simulink model "minimum_snap_trajectory"  (R2021a)
settings: Solver=VariableStepAuto  StartTime=0.0  StopTime=T_s  RelTol=1e-3
values from neighbouring files (symbols this model uses):
  a_x = x(1,1:(length(x)-1))    [Linearized_model.m]    (also in Linearized_model_motor_dynamics.m)
  a_y = y(1,1:(length(y)-1))    [Linearized_model.m]    (also in Linearized_model_motor_dynamics.m)
  a_z = z(1,1:(length(z)-1))    [Linearized_model.m]    (also in Linearized_model_motor_dynamics.m)
  b_x = x(1,2:length(x))    [Linearized_model.m]    (also in Linearized_model_motor_dynamics.m)
  b_y = y(1,2:length(y))    [Linearized_model.m]    (also in Linearized_model_motor_dynamics.m)
  b_z = z(1,2:length(z))    [Linearized_model.m]    (also in Linearized_model_motor_dynamics.m)
  T_r = zeros(1, length(T))    [Linearized_model.m]    (also in Linearized_model_motor_dynamics.m)
  T_s = sum(T)    [Linearized_model.m]    (also in Linearized_model_motor_dynamics.m)
undefined symbols (not defined in the file or in its folder): a_phi, a_si, a_theta, b_phi, b_si, b_theta
settings Model: Creator=Traveler  LastModifiedBy=Traveler

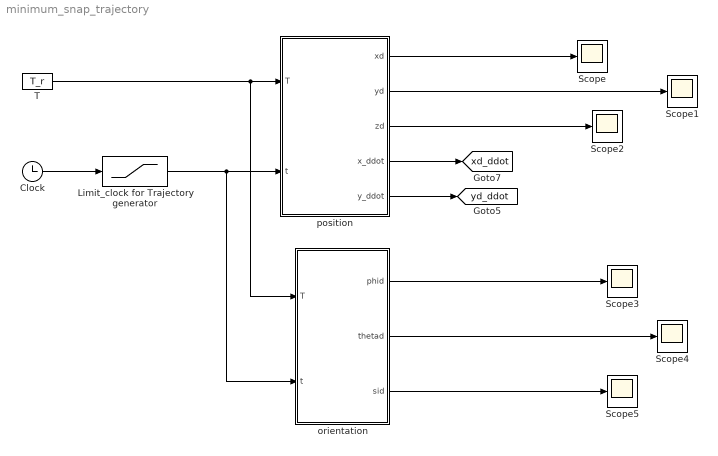
== system minimum_snap_trajectory ==
  Clock : Clock
  Limit_clock for Trajectory generator : Saturate  UpperLimit=T_s  LowerLimit=0
  Scope{,1..5} (6 alike) : Scope
  T : Constant  Value=T_r
  orientation : Subsystem
  position : Subsystem
  tag scope: xd_ddot=global, yd_ddot=global
  wires:
  position/5(y_ddot) -> [yd_ddot]
  T/1 -> orientation/1(T), position/1(T)
  Clock/1 -> Limit_clock for Trajectory generator/1
  orientation/2(thetad) -> Scope4/1
  position/2(yd) -> Scope1/1
  Limit_clock for Trajectory generator/1 -> orientation/2(t), position/2(t)
  position/3(zd) -> Scope2/1
  position/1(xd) -> Scope/1
  position/4(x_ddot) -> [xd_ddot]
  orientation/1(phid) -> Scope3/1
  orientation/3(sid) -> Scope5/1

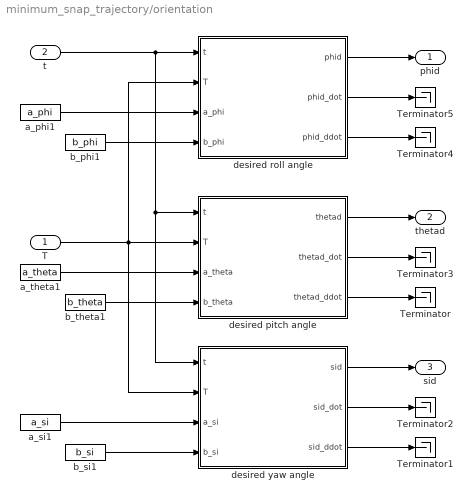
== system minimum_snap_trajectory/orientation ==
  T : Inport
  t : Inport  Port=2
  " desired pitch angle" : MATLAB Function  TreatAsAtomicUnit=on
  Terminator{,1..5} (6 alike) : Terminator
  a_phi1 : Constant  Value=a_phi
  a_si1 : Constant  Value=a_si
  a_theta1 : Constant  Value=a_theta
  b_phi1 : Constant  Value=b_phi
  b_si1 : Constant  Value=b_si
  b_theta1 : Constant  Value=b_theta
  desired roll angle : MATLAB Function  TreatAsAtomicUnit=on
  desired yaw angle : MATLAB Function  TreatAsAtomicUnit=on
  phid : Outport
  thetad : Outport  Port=2
  sid : Outport  Port=3
  wires:
  desired roll angle/1(phid) -> phid/1
  desired roll angle/2(phid_dot) -> Terminator5/1
  desired roll angle/3(phid_ddot) -> Terminator4/1
  " desired pitch angle"/3(thetad_ddot) -> Terminator/1
  " desired pitch angle"/2(thetad_dot) -> Terminator3/1
  " desired pitch angle"/1(thetad) -> thetad/1
  desired yaw angle/1(sid) -> sid/1
  desired yaw angle/2(sid_dot) -> Terminator2/1
  desired yaw angle/3(sid_ddot) -> Terminator1/1
  a_phi1/1 -> desired roll angle/3(a_phi)
  b_phi1/1 -> desired roll angle/4(b_phi)
  a_theta1/1 -> " desired pitch angle"/3(a_theta)
  b_theta1/1 -> " desired pitch angle"/4(b_theta)
  a_si1/1 -> desired yaw angle/3(a_si)
  b_si1/1 -> desired yaw angle/4(b_si)
  T/1 -> desired roll angle/2(T), " desired pitch angle"/2(T), desired yaw angle/2(T)
  t/1 -> desired yaw angle/1(t), " desired pitch angle"/1(t), desired roll angle/1(t)

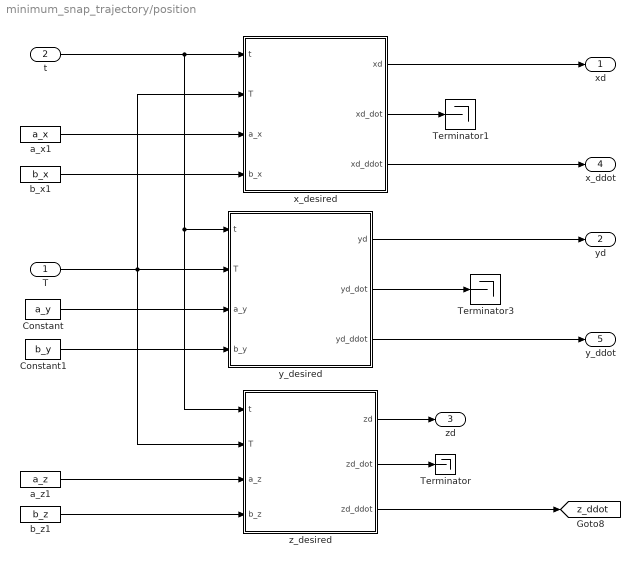
== system minimum_snap_trajectory/position ==
  T : Inport
  t : Inport  Port=2
  " z_desired" : MATLAB Function  TreatAsAtomicUnit=on
  Constant : Constant  Value=a_y
  Constant1 : Constant  Value=b_y
  Terminator : Terminator
  Terminator1 : Terminator
  Terminator3 : Terminator
  a_x1 : Constant  Value=a_x
  a_z1 : Constant  Value=a_z
  b_x1 : Constant  Value=b_x
  b_z1 : Constant  Value=b_z
  x_desired : MATLAB Function  TreatAsAtomicUnit=on
  y_desired : MATLAB Function  TreatAsAtomicUnit=on
  xd : Outport
  yd : Outport  Port=2
  zd : Outport  Port=3
  x_ddot : Outport  Port=4
  y_ddot : Outport  Port=5
  tag scope: z_ddot=global
  wires:
  y_desired/1(yd) -> yd/1
  T/1 -> x_desired/2(T), y_desired/2(T), " z_desired"/2(T)
  a_x1/1 -> x_desired/3(a_x)
  b_x1/1 -> x_desired/4(b_x)
  Constant/1 -> y_desired/3(a_y)
  Constant1/1 -> y_desired/4(b_y)
  a_z1/1 -> " z_desired"/3(a_z)
  b_z1/1 -> " z_desired"/4(b_z)
  " z_desired"/2(zd_dot) -> Terminator/1
  x_desired/2(xd_dot) -> Terminator1/1
  y_desired/2(yd_dot) -> Terminator3/1
  t/1 -> x_desired/1(t), y_desired/1(t), " z_desired"/1(t)
  " z_desired"/3(zd_ddot) -> [z_ddot]
  " z_desired"/1(zd) -> zd/1
  y_desired/3(yd_ddot) -> y_ddot/1
  x_desired/3(xd_ddot) -> x_ddot/1
  x_desired/1(xd) -> xd/1

== matlab function minimum_snap_trajectory/orientation/ desired pitch angle ==
  data: t input; T input; thetad output; thetad_dot output; thetad_ddot output; a_theta input; b_theta input
function [thetad,thetad_dot,thetad_ddot] = fcn(t,T,a_theta,b_theta)
T0 = 0; % Initialize T0
Tf = 0; % Initialize Tf
a = 0;  % Initialize a
b = 0;  % Initialize b

for i = 1:length(T)
    if (i == 1 && t <= T(i))
        Tf = T(i);
        a = a_theta(i);
        b = b_theta(i);
        break;
    elseif (i > 1 && t > T(i-1) && t <= T(i))
        T0 = T(i-1);
        Tf = T(i);
        a = a_theta(i);
        b = b_theta(i);
        break;
    end
end
if (t > T(end-1)) % Handle the case where t is greater than the last interval
    T0 = T(end-1);
    Tf = T(end);
    a = a_theta(end);
    b = b_theta(end);
end
B=[a;b;0;0;0;0];
A=[T0^5     T0^4     T0^3    T0^2  T0^1  1;
   Tf^5     Tf^4     Tf^3    Tf^2  Tf^1  1;
   5*T0^4   4*T0^3   3*T0^2  2*T0  1     0;
   5*Tf^4   4*Tf^3   3*Tf^2  2*Tf  1     0;
   20*T0^3  12*T0^2  6*T0    2     0     0;
   20*Tf^3  12*Tf^2  6*Tf    2     0     0];
C=A\B;
thetad=C(1,1)*t^5 + C(2,1)*t^4 + C(3,1)*t^3 + C(4,1)*t^2 + C(5,1)*t + C(6,1);
thetad_dot=5*C(1,1)*t^4  + 4*C(2,1)*t^3 + 3*C(3,1)*t^2 + 2*C(4,1)*t + C(5,1);
thetad_ddot=20*C(1,1)*t^3  + 12*C(2,1)*t^2 + 6*C(3,1)*t + 2*C(4,1);
end

== matlab function minimum_snap_trajectory/orientation/desired roll angle ==
  data: t input; T input; phid output; phid_dot output; phid_ddot output; a_phi input; b_phi input
function [phid,phid_dot,phid_ddot] = fcn(t,T,a_phi,b_phi)
T0 = 0; % Initialize T0
Tf = 0; % Initialize Tf
a = 0;  % Initialize a
b = 0;  % Initialize b

for i = 1:length(T)
    if (i == 1 && t <= T(i))
        Tf = T(i);
        a = a_phi(i);
        b = b_phi(i);
        break;
    elseif (i > 1 && t > T(i-1) && t <= T(i))
        T0 = T(i-1);
        Tf = T(i);
        a = a_phi(i);
        b = b_phi(i);
        break;
    end
end
if (t > T(end-1)) % Handle the case where t is greater than the last interval
    T0 = T(end-1);
    Tf = T(end);
    a = a_phi(end);
    b = b_phi(end);
end
B=[a;b;0;0;0;0];
A=[T0^5     T0^4     T0^3    T0^2  T0^1  1;
   Tf^5     Tf^4     Tf^3    Tf^2  Tf^1  1;
   5*T0^4   4*T0^3   3*T0^2  2*T0  1     0;
   5*Tf^4   4*Tf^3   3*Tf^2  2*Tf  1     0;
   20*T0^3  12*T0^2  6*T0    2     0     0;
   20*Tf^3  12*Tf^2  6*Tf    2     0     0];
C=A\B;
phid=C(1,1)*t^5 + C(2,1)*t^4 + C(3,1)*t^3 + C(4,1)*t^2 + C(5,1)*t + C(6,1);
phid_dot=5*C(1,1)*t^4  + 4*C(2,1)*t^3 + 3*C(3,1)*t^2 + 2*C(4,1)*t + C(5,1);
phid_ddot=20*C(1,1)*t^3  + 12*C(2,1)*t^2 + 6*C(3,1)*t + 2*C(4,1);
end

== matlab function minimum_snap_trajectory/orientation/desired yaw angle ==
  data: t input; T input; sid output; sid_dot output; sid_ddot output; a_si input; b_si input
function [sid,sid_dot,sid_ddot] = fcn(t,T,a_si,b_si)
T0 = 0; % Initialize T0
Tf = 0; % Initialize Tf
a = 0;  % Initialize a
b = 0;  % Initialize b

for i = 1:length(T)
    if (i == 1 && t <= T(i))
        Tf = T(i);
        a = a_si(i);
        b = b_si(i);
        break;
    elseif (i > 1 && t > T(i-1) && t <= T(i))
        T0 = T(i-1);
        Tf = T(i);
        a = a_si(i);
        b = b_si(i);
        break;
    end
end
if (t > T(end-1)) % Handle the case where t is greater than the last interval
    T0 = T(end-1);
    Tf = T(end);
    a = a_si(end);
    b = b_si(end);
end
B=[a;b;0;0;0;0];
A=[T0^5     T0^4     T0^3    T0^2  T0^1  1;
   Tf^5     Tf^4     Tf^3    Tf^2  Tf^1  1;
   5*T0^4   4*T0^3   3*T0^2  2*T0  1     0;
   5*Tf^4   4*Tf^3   3*Tf^2  2*Tf  1     0;
   20*T0^3  12*T0^2  6*T0    2     0     0;
   20*Tf^3  12*Tf^2  6*Tf    2     0     0];
C=A\B;
sid=C(1,1)*t^5 + C(2,1)*t^4 + C(3,1)*t^3 + C(4,1)*t^2 + C(5,1)*t + C(6,1);
sid_dot=5*C(1,1)*t^4  + 4*C(2,1)*t^3 + 3*C(3,1)*t^2 + 2*C(4,1)*t + C(5,1);
sid_ddot=20*C(1,1)*t^3  + 12*C(2,1)*t^2 + 6*C(3,1)*t + 2*C(4,1);
end

== matlab function minimum_snap_trajectory/position/ z_desired ==
  data: t input; T input; zd output; zd_dot output; zd_ddot output; a_z input; b_z input
function [zd,zd_dot,zd_ddot] = fcn(t,T,a_z,b_z)
T0 = 0; % Initialize T0
Tf = 0; % Initialize Tf
a = 0;  % Initialize a
b = 0;  % Initialize b

for i = 1:length(T)
    if (i == 1 && t <= T(i))
        Tf = T(i);
        a = a_z(i);
        b = b_z(i);
        break;
    elseif (i > 1 && t > T(i-1) && t <= T(i))
        T0 = T(i-1);
        Tf = T(i);
        a = a_z(i);
        b = b_z(i);
        break;
    end
end
if (t > T(end-1)) % Handle the case where t is greater than the last interval
    T0 = T(end-1);
    Tf = T(end);
    a = a_z(end);
    b = b_z(end);
end
B=[a;b;0;0;0;0];
A=[T0^5     T0^4     T0^3    T0^2  T0^1  1;
   Tf^5     Tf^4     Tf^3    Tf^2  Tf^1  1;
   5*T0^4   4*T0^3   3*T0^2  2*T0  1     0;
   5*Tf^4   4*Tf^3   3*Tf^2  2*Tf  1     0;
   20*T0^3  12*T0^2  6*T0    2     0     0;
   20*Tf^3  12*Tf^2  6*Tf    2     0     0];
C=A\B;
zd=C(1,1)*t^5 + C(2,1)*t^4 + C(3,1)*t^3 + C(4,1)*t^2 + C(5,1)*t + C(6,1);
zd_dot=5*C(1,1)*t^4  + 4*C(2,1)*t^3 + 3*C(3,1)*t^2 + 2*C(4,1)*t + C(5,1);
zd_ddot=20*C(1,1)*t^3  + 12*C(2,1)*t^2 + 6*C(3,1)*t + 2*C(4,1);
end

== matlab function minimum_snap_trajectory/position/x_desired ==
  data: t input; T input; xd output; xd_dot output; xd_ddot output; a_x input; b_x input
function [xd,xd_dot,xd_ddot] = fcn(t,T,a_x,b_x)
T0 = 0; % Initialize T0
Tf = 0; % Initialize Tf
a = 0;  % Initialize a
b = 0;  % Initialize b

for i = 1:length(T)
    if (i == 1 && t <= T(i))
        Tf = T(i);
        a = a_x(i);
        b = b_x(i);
        break;
    elseif (i > 1 && t > T(i-1) && t <= T(i))
        T0 = T(i-1);
        Tf = T(i);
        a = a_x(i);
        b = b_x(i);
        break;
    end
end
if (t > T(end-1)) % Handle the case where t is greater than the last interval
    T0 = T(end-1);
    Tf = T(end);
    a = a_x(end);
    b = b_x(end);
end
B=[a;b;0;0;0;0];
A=[T0^5     T0^4     T0^3    T0^2  T0^1  1;
   Tf^5     Tf^4     Tf^3    Tf^2  Tf^1  1;
   5*T0^4   4*T0^3   3*T0^2  2*T0  1     0;
   5*Tf^4   4*Tf^3   3*Tf^2  2*Tf  1     0;
   20*T0^3  12*T0^2  6*T0    2     0     0;
   20*Tf^3  12*Tf^2  6*Tf    2     0     0];
C=A\B;
xd=C(1,1)*t^5 + C(2,1)*t^4 + C(3,1)*t^3 + C(4,1)*t^2 + C(5,1)*t + C(6,1);
xd_dot=5*C(1,1)*t^4  + 4*C(2,1)*t^3 + 3*C(3,1)*t^2 + 2*C(4,1)*t + C(5,1);
xd_ddot=20*C(1,1)*t^3  + 12*C(2,1)*t^2 + 6*C(3,1)*t + 2*C(4,1);
end

== matlab function minimum_snap_trajectory/position/y_desired ==
  data: t input; T input; yd output; yd_dot output; yd_ddot output; a_y input; b_y input
function [yd,yd_dot,yd_ddot] = fcn(t,T,a_y,b_y)
T0 = 0; % Initialize T0
Tf = 0; % Initialize Tf
a = 0;  % Initialize a
b = 0;  % Initialize b

for i = 1:length(T)
    if (i == 1 && t <= T(i))
        Tf = T(i);
        a = a_y(i);
        b = b_y(i);
        break;
    elseif (i > 1 && t > T(i-1) && t <= T(i))
        T0 = T(i-1);
        Tf = T(i);
        a = a_y(i);
        b = b_y(i);
        break;
    end
end
if (t > T(end-1)) % Handle the case where t is greater than the last interval
    T0 = T(end-1);
    Tf = T(end);
    a = a_y(end);
    b = b_y(end);
end
B=[a;b;0;0;0;0];
A=[T0^5     T0^4     T0^3    T0^2  T0^1  1;
   Tf^5     Tf^4     Tf^3    Tf^2  Tf^1  1;
   5*T0^4   4*T0^3   3*T0^2  2*T0  1     0;
   5*Tf^4   4*Tf^3   3*Tf^2  2*Tf  1     0;
   20*T0^3  12*T0^2  6*T0    2     0     0;
   20*Tf^3  12*Tf^2  6*Tf    2     0     0];
C=A\B;
yd=C(1,1)*t^5 + C(2,1)*t^4 + C(3,1)*t^3 + C(4,1)*t^2 + C(5,1)*t + C(6,1);
yd_dot=5*C(1,1)*t^4  + 4*C(2,1)*t^3 + 3*C(3,1)*t^2 + 2*C(4,1)*t + C(5,1);
yd_ddot=20*C(1,1)*t^3  + 12*C(2,1)*t^2 + 6*C(3,1)*t + 2*C(4,1);
end
